simulink model "CL_NL_DH_GUIA_Original"  (R2025b)
settings: Solver=ode4  StartTime=0.0  StopTime=200  FixedStep=Ts  RelTol=1e-3
values from neighbouring files (symbols this model uses):
  alpha_prot = deg2rad(16)    [guiagem_NL.m]
  att_alt = 0    [guiagem_NL.m]
  de_trim = U_trim(2)    [guiagem_NL.m]
  h0 = 600    [guiagem_NL.m]
  h_ref0 = h0    (= 600)    [guiagem_NL.m]
  i = find([Plantas.Ve] == VT_missao & [Plantas.He] == 600, 1)    [guiagem_NL.m]
  K_bank_guia = 0.1975    [guiagem_NL.m]
  phi_max_guia = deg2rad(20)    [guiagem_NL.m]
  phi_psi = 0    [guiagem_NL.m]
  prot_on = 0    [guiagem_NL.m]
  sat_surf_rad = deg2rad(sat_deg)    [guiagem_NL.m]
  surfaces = 24    [guiagem_NL.m]
  U_trim = double(Plantas(i).Ue(1:4))    [guiagem_NL.m]
  VT_ref0 = VT_missao    [guiagem_NL.m]
  VT_Throttle = 1    [guiagem_NL.m]
  WPs = [ 256    0  600  15 ... (first row only)    [guiagem_NL.m]
  xi_alt0 = double(Plantas(i).Xe(8)) / double(GintLong_Alt{i})    [guiagem_NL.m]
undefined symbols (not defined in the file or in its folder): act, eng, Plantas, R_accept, TrimInput
libraries: simulink_extras x10, simulink x1
settings Model: SimulationMode=accelerator  Creator=mirko  LastModifiedBy=mirko

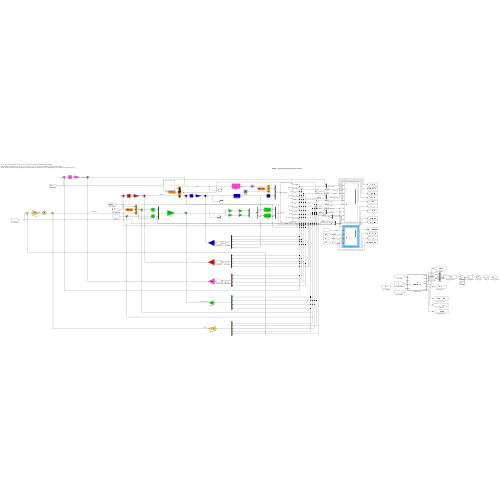
[thumbnail: Simulink's stored preview of the top-level diagram]
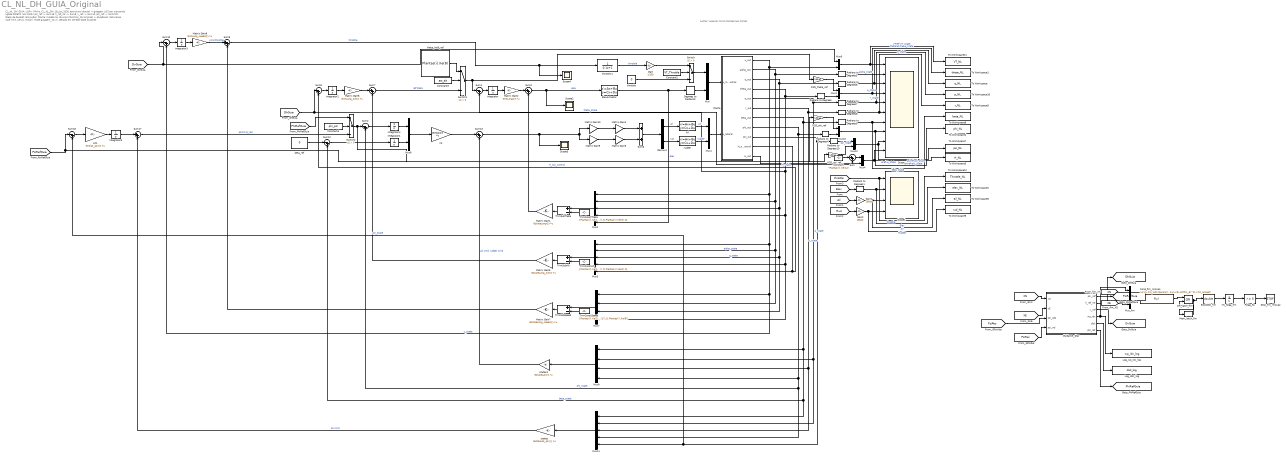
== system CL_NL_DH_GUIA_Original ==
  note: Author: Huascar Mirko Montecinos Cortez
  note: CL_NL_DH_GUIA: LQRy (Mirko, CL_NL_DH_18_jun_2026, estrutura intacta) + guiagem LOS por waypoints
      | ligada DIRETO nos holds (psi_ref -> Sum18, h_ref_rel -> Sum8, v_ref -> Sum10, phi_ref -> Switch2). Steps de doublet removidos.
      | Planta: modelo NL da Ana (sfunction_DH original) + atuadores (saturacao, rate limit, servo, motor). Rode guiagem_NL.m. Gerado em 03-Sep-2026 14:46:32.
  Ail : StateSpace  A=-surfaces  B=surfaces  D=0  InitialCondition=0
  Bool2Dbl_fim : DataTypeConversion  OutDataTypeStr=double  SaturateOnIntegerOverflow=off  RndMeth=Floor
  Cond_fim_missao : Fcn  Expr=(u(1)>=N_WPs)&&(sqrt((u(2)-WPfim_N)^2+(u(3)-WPfim_E)^2)<=R_accept)
  Constant : Constant  Value=-Plantas(i).Xe(12)
  Constant2 : Constant  Value=VT_Throttle
  Constant3 : Constant  Value=att_alt
  Constant4 : Constant  Value=phi_psi
  Degrees to Radians3 : simulink_extras/Transformations/Degrees to Radians
  Demux4 : Demux  Outputs=2
      settings: DisplayOption=none
  ElevActuator : StateSpace  A=-surfaces  B=surfaces  D=0  InitialCondition=Plantas(i).Ue(2)
  Folga_5s : simulink/Logic and Bit Operations/Compare To Constant  relop=>=  const=5  OutDataTypeStr=boolean
  Gain : Gain  Gain=1/100
  Gain1 : Gain  Gain=180/pi
  Gain2 : Gain  Gain=180/pi
  Guidance_Star : MATLAB Function  TreatAsAtomicUnit=on
  Int_folga_fim : Integrator
  Integrator{,1,3..5} (5 alike) : Integrator
  Integrator2 : Integrator  InitialCondition=xi_alt0
  Log_dist_log : ToWorkspace  VariableName=dist_log  SampleTime=-1
  Log_wp_idx_log : ToWorkspace  VariableName=wp_idx_log  SampleTime=-1
  Matrix Gain1 : Gain  Gain=GstateLong{i}  Multiplication=Matrix(K*u)  SaturateOnIntegerOverflow=on  OutDataTypeStr=Inherit: Same as input  ParamDataTypeStr=Inherit: Same as input
  Matrix Gain10 : Gain  Gain=[1 0]  Multiplication=Matrix(K*u)  SaturateOnIntegerOverflow=on  OutDataTypeStr=Inherit: Same as input  ParamDataTypeStr=Inherit: Same as input
  Matrix Gain2 : Gain  Gain=GintLong{i}  Multiplication=Matrix(K*u)  SaturateOnIntegerOverflow=on  OutDataTypeStr=Inherit: Same as input  ParamDataTypeStr=Inherit: Same as input
  Matrix Gain3 : Gain  Gain=[0 1]'  Multiplication=Matrix(K*u)  SaturateOnIntegerOverflow=on  OutDataTypeStr=Inherit: Same as input  ParamDataTypeStr=Inherit: Same as input
  Matrix Gain4 : Gain  Gain=[1 0]'  Multiplication=Matrix(K*u)  SaturateOnIntegerOverflow=on  OutDataTypeStr=Inherit: Same as input  ParamDataTypeStr=Inherit: Same as input
  Matrix Gain5 : Gain  Gain=GstateLong_Alt{i}  Multiplication=Matrix(K*u)  SaturateOnIntegerOverflow=on  OutDataTypeStr=Inherit: Same as input  ParamDataTypeStr=Inherit: Same as input
  Matrix Gain6 : Gain  Gain=GintLong_Alt{i}  Multiplication=Matrix(K*u)  SaturateOnIntegerOverflow=on  OutDataTypeStr=Inherit: Same as input  ParamDataTypeStr=Inherit: Same as input
  Matrix Gain7 : Gain  Gain=GstateLong_speed{i}  Multiplication=Matrix(K*u)  SaturateOnIntegerOverflow=on  OutDataTypeStr=Inherit: Same as input  ParamDataTypeStr=Inherit: Same as input
  Matrix Gain8 : Gain  Gain=GintLong_speed{i}  Multiplication=Matrix(K*u)  SaturateOnIntegerOverflow=on  OutDataTypeStr=Inherit: Same as input  ParamDataTypeStr=Inherit: Same as input
  Matrix Gain9 : Gain  Gain=[0 1]  Multiplication=Matrix(K*u)  SaturateOnIntegerOverflow=on  OutDataTypeStr=Inherit: Same as input  ParamDataTypeStr=Inherit: Same as input
  Mem_latch_fim : Memory
  Mux{,1,3..4,6,8,10,12} (8 alike) : Mux  Inputs=2
  Mux11 : Mux  Inputs=5
  Mux2 : Mux  Inputs=5
  Mux5 : Mux  Inputs=5
  Mux7 : Mux
  Mux9 : Mux
  Mux_fim : Mux  Inputs=3
  OR_latch_fim : Logic  Operator=OR  AllPortsSameDT=off  OutDataTypeStr=boolean
  Planta : Subsystem
  R2D_phi_ref : Gain  Gain=180/pi
  R2D_psi_ref : Gain  Gain=180/pi
  R2D_theta_ref : Gain  Gain=180/pi
  Radians to Degrees{,1,4..10} (9 alike) : simulink_extras/Transformations/Radians to Degrees
  Scope : Scope  NumInputPorts=10
      settings: ActiveDisplayString=10  ActiveDisplayYMinimum=599.95100767099655  ActiveDisplayYMaximum=600.03459621742491
  Scope1 : Scope  NumInputPorts=4
      settings: ActiveDisplayString=4  ActiveDisplayYMinimum=-3.1238215479894382  ActiveDisplayYMaximum=4.435550961328742
  Scope2 : Scope
      settings: ActiveDisplayYMinimum=-1.3531942213324573  ActiveDisplayYMaximum=0.61662907005096645  DataLoggingVariableName=ScopeData2
  Scope3 : Scope
      settings: ActiveDisplayYMinimum=-0.008953837623387962  ActiveDisplayYMaximum=0.0080763644870395709  DataLoggingVariableName=ScopeData3
  Scope4 : Scope
      settings: ActiveDisplayYMinimum=-268.65761065429206  ActiveDisplayYMaximum=1519.894817061396  DataLoggingVariableName=ScopeData4
  Stop_fim_missao : Stop
  Sum{,3,7,9} (4 alike) : Sum  Inputs=|++
  Sum1 : Sum  Inputs=|-+
  Sum10 : Sum  Inputs=|-+
  Sum12 : Sum  Inputs=|-+  SaturateOnIntegerOverflow=on
  Sum13 : Sum  Inputs=|++  SaturateOnIntegerOverflow=on
  Sum17 : Sum  Inputs=|++  SaturateOnIntegerOverflow=on
  Sum18 : Sum  Inputs=|-+  SaturateOnIntegerOverflow=on
  Sum2 : Sum  Inputs=|-+  SaturateOnIntegerOverflow=on
  Sum6 : Sum  Inputs=2  SaturateOnIntegerOverflow=on
  Sum8 : Sum  Inputs=|-+
  Switch : Switch  Criteria=u2 > Threshold  SaturateOnIntegerOverflow=off  InputSameDT=off
  Switch1 : Switch  Criteria=u2 > Threshold  SaturateOnIntegerOverflow=off  InputSameDT=off
  Switch2 : Switch  Criteria=u2 > Threshold  SaturateOnIntegerOverflow=off  InputSameDT=off
  To Workspace : ToWorkspace  VariableName=q_NL  SaveFormat=Structure With Time  SampleTime=-1
  To Workspace1 : ToWorkspace  VariableName=theta_NL  SaveFormat=Structure With Time  SampleTime=-1
  To Workspace10 : ToWorkspace  VariableName=p_NL  SaveFormat=Structure With Time  SampleTime=-1
  To Workspace11 : ToWorkspace  VariableName=VT_NL  SaveFormat=Structure With Time  SampleTime=-1
  To Workspace12 : ToWorkspace  VariableName=Throttle_NL  SaveFormat=Structure With Time  SampleTime=-1
  To Workspace2 : ToWorkspace  VariableName=elev_NL  SaveFormat=Structure With Time  SampleTime=-1
  To Workspace3 : ToWorkspace  VariableName=H_NL  SaveFormat=Structure With Time  SampleTime=-1
  To Workspace4 : ToWorkspace  VariableName=phi_NL  SaveFormat=Structure With Time  SampleTime=-1
  To Workspace5 : ToWorkspace  VariableName=r_NL  SaveFormat=Structure With Time  SampleTime=-1
  To Workspace6 : ToWorkspace  VariableName=ail_NL  SaveFormat=Structure With Time  SampleTime=-1
  To Workspace7 : ToWorkspace  VariableName=psi_NL  SaveFormat=Structure With Time  SampleTime=-1
  To Workspace8 : ToWorkspace  VariableName=beta_NL  SaveFormat=Structure With Time  SampleTime=-1
  To Workspace9 : ToWorkspace  VariableName=rud_NL  SaveFormat=Structure With Time  SampleTime=-1
  TrimConstAlt : Constant  Value=[Plantas(i).Xe(1); atan(Plantas(i).Xe(3)/Plantas(i).Xe(1)); 0; Plantas(i).Xe(8); 0]  VectorParams1D=off
  TrimConstSpeed : Constant  Value=[Plantas(i).Xe(1); atan(Plantas(i).Xe(3)/Plantas(i).Xe(1)); 0; Plantas(i).Xe(8)]  VectorParams1D=off
  TrimConstTheta : Constant  Value=[Plantas(i).Xe(1); atan(Plantas(i).Xe(3)/Plantas(i).Xe(1)); 0; Plantas(i).Xe(8); 0]  VectorParams1D=off
  TrimSubAlt : Sum  Inputs=+-
  TrimSubSpeed : Sum  Inputs=+-
  TrimSubTheta : Sum  Inputs=+-
  beta_ref : Constant  Value=0
  int : Gain  Gain=Gintlat{i}  Multiplication=Matrix(K*u)  SaturateOnIntegerOverflow=on  OutDataTypeStr=Inherit: Same as input  ParamDataTypeStr=Inherit: Same as input
  int1 : Gain  Gain=Gintlat_psi{i}  Multiplication=Matrix(K*u)  SaturateOnIntegerOverflow=on  OutDataTypeStr=Inherit: Same as input  ParamDataTypeStr=Inherit: Same as input
  rudder : StateSpace  A=-surfaces  B=surfaces  D=0  InitialCondition=0
  states : Gain  Gain=GstateLat_psi{i}  Multiplication=Matrix(K*u)  SaturateOnIntegerOverflow=on  OutDataTypeStr=Inherit: Same as input  ParamDataTypeStr=Inherit: Same as input
  states1 : Gain  Gain=GstateLat{i}  Multiplication=Matrix(K*u)  SaturateOnIntegerOverflow=on  OutDataTypeStr=Inherit: Same as input  ParamDataTypeStr=Inherit: Same as input
  theta_hold_ref : Constant  Value=Plantas(i).Xe(8)
  throttle : Constant  Value=0
  throttle 1 : TransferFcn  Denominator=[0.1 1]
  tag scope: DhGuia=global, DvGuia=global, PhiRefGuia=global, PsiRefGuia=global
  wires:
  Mux/1 -> Planta/1(u_longitudinal)
  Mux1/1 -> Planta/2(u_lateral)
  Matrix Gain1/1 -> Sum3/2
  Matrix Gain2/1 -> Sum3/1
  Integrator/1 -> Matrix Gain2/1
  Sum1/1 -> Integrator/1
  Sum3/1 -> Scope2/1, ElevActuator/1  "elev"
  Planta/1(u_out) -> Mux6/2, Mux7/1, Sum10/2, Mux5/1, Mux2/1  "u_state"
  Planta/2(alpha_out) -> Mux7/2, Mux5/2, Mux2/2, Radians to Degrees5/1  "alpha_state"
  Planta/3(q_out) -> Mux7/3, Mux5/3, Mux2/3, Radians to Degrees6/1  "q_state"
  Planta/4(theta_out) -> Mux7/4, Mux5/4, Mux2/4, Sum1/2, Radians to Degrees/1  "theta_state"
  Planta/5(p_out) -> Radians to Degrees7/1, Mux9/2, Mux11/2  "p_state"
  Planta/6(r_out) -> Radians to Degrees8/1, Mux9/3, Mux11/3  "r_state"
  Planta/7(beta_out) -> Radians to Degrees9/1, Mux11/1, Sum12/2, Mux9/1  "beta_state"
  Planta/8(phi_out) -> Radians to Degrees4/1, Mux11/4, Sum2/2, Mux9/4  "phi_state"
  Planta/9(psi_out) -> Mux11/5, Sum18/2, Radians to Degrees10/1  "psi_state"
  Planta/10(H_out_control) -> Mux5/5, Sum8/2  "H_out_control"
  Mux3/1 -> To Workspace1/1, Scope/4  "thetaref-theta_state"
  Radians to Degrees/1 -> Mux3/2
  Matrix Gain5/1 -> Sum7/2
  Sum8/1 -> Integrator2/1
  Sum7/1 -> Switch1/3  "ref theta"
  Matrix Gain6/1 -> Sum7/1
  Integrator2/1 -> Matrix Gain6/1
  Mux4/1 -> Scope/10, To Workspace3/1  "Href-H_state"
  Constant/1 -> Sum/1
  Sum/1 -> Mux4/1
  Radians to Degrees1/1 -> Scope1/2, To Workspace2/1  "Elev"
  Gain1/1 -> Scope1/3, To Workspace6/1  "Ail"
  Gain2/1 -> Scope1/4, To Workspace9/1  "Rudder"
  Sum10/1 -> Integrator3/1
  Matrix Gain7/1 -> Sum9/2
  Integrator3/1 -> Matrix Gain8/1
  Matrix Gain8/1 -> Sum9/1  "cmd throttle"
  [Elev] -> Radians to Degrees1/1
  [Ail] -> Gain1/1
  [Rud] -> Gain2/1
  [throttle] -> To Workspace12/1, Scope1/1  "throttle"
  Sum9/1 -> Scope4/1, throttle 1/1  "throttle"
  Mux6/1 -> To Workspace11/1, Scope/1  "VTref-VT_state"
  Matrix Gain9/1 -> Matrix Gain3/1
  Matrix Gain10/1 -> Matrix Gain4/1
  Matrix Gain4/1 -> Sum6/1
  Sum13/1 -> Scope3/1, Matrix Gain9/1, Matrix Gain10/1
  Matrix Gain3/1 -> Sum6/2
  Sum6/1 -> Demux4/1
  Demux4/2 -> rudder/1  "rud"
  Demux4/1 -> Ail/1  "ail"
  int/1 -> Sum13/1
  Mux8/1 -> int/1
  Sum12/1 -> Integrator1/1
  Integrator4/1 -> Mux8/1
  Integrator1/1 -> Mux8/2
  Sum2/1 -> Integrator4/1
  Mux9/1 -> states1/1
  states1/1 -> Sum13/2  "ail cmd, rudder cmd"
  Mux10/1 -> To Workspace4/1, Scope/8  "phiref-phi_state"
  Radians to Degrees4/1 -> Mux10/2
  throttle/1 -> Switch/3
  Radians to Degrees5/1 -> Scope/2  "alpha_state"
  Radians to Degrees6/1 -> To Workspace/1, Scope/3  "q_state"
  Radians to Degrees7/1 -> To Workspace10/1, Scope/5  "p_state"
  Radians to Degrees8/1 -> Scope/6, To Workspace5/1  "r_state"
  Radians to Degrees9/1 -> Scope/7, To Workspace8/1  "beta_state"
  Degrees to Radians3/1 -> Mux/2
  Gain/1 -> Switch/1
  Mux12/1 -> To Workspace7/1, Scope/9  "psiref-psi_state"
  Planta/11(H_out) -> Mux4/2  "H_state"
  Mux11/1 -> states/1
  Sum18/1 -> int1/1
  Integrator5/1 -> Sum17/1
  int1/1 -> Integrator5/1
  Sum17/1 -> Switch2/3  "psiCmd_rad"
  states/1 -> Sum17/2  "ail cmd"
  Switch2/1 -> Sum2/1, R2D_phi_ref/1
  Radians to Degrees10/1 -> Mux12/1  "psi_state"
  Constant2/1 -> Switch/2
  Constant3/1 -> Switch1/2
  Constant4/1 -> Switch2/2
  Mux7/1 -> TrimSubSpeed/1
  TrimConstSpeed/1 -> TrimSubSpeed/2
  TrimSubSpeed/1 -> Matrix Gain7/1
  Mux2/1 -> TrimSubTheta/1
  TrimConstTheta/1 -> TrimSubTheta/2
  TrimSubTheta/1 -> Matrix Gain1/1
  Mux5/1 -> TrimSubAlt/1
  TrimConstAlt/1 -> TrimSubAlt/2
  TrimSubAlt/1 -> Matrix Gain5/1
  throttle 1/1 -> Gain/1  "throttle"
  rudder/1 -> Mux1/2  "rudder"
  Ail/1 -> Mux1/1  "Ail"
  ElevActuator/1 -> Degrees to Radians3/1, Mux2/5  "elev"
  Switch/1 -> Mux/1
  [XN] -> Guidance_Star/1(xN)
  [PsiRel] -> Guidance_Star/4(psi_rel)
  [PsiAbs] -> Guidance_Star/3(psi_abs)
  [XE] -> Guidance_Star/2(xE)
  Guidance_Star/1(psi_ref) -> [PsiRefGuia]
  Guidance_Star/2(h_ref_rel) -> [DhGuia]
  Guidance_Star/3(v_ref) -> [DvGuia]
  Guidance_Star/4(wp_idx) -> Log_wp_idx_log/1, Mux_fim/1
  Guidance_Star/5(dist) -> Log_dist_log/1
  Guidance_Star/6(phi_ref) -> [PhiRefGuia]
  [PsiRefGuia] -> Sum18/1, R2D_psi_ref/1
  [DhGuia] -> Sum8/1, Sum/2
  [DvGuia] -> Sum10/1, Mux6/1
  [PhiRefGuia] -> Switch2/1
  theta_hold_ref/1 -> Switch1/1
  Switch1/1 -> Sum1/1, R2D_theta_ref/1
  beta_ref/1 -> Sum12/1
  R2D_theta_ref/1 -> Mux3/1
  R2D_psi_ref/1 -> Mux12/2
  R2D_phi_ref/1 -> Mux10/1
  [XN] -> Mux_fim/2
  [XE] -> Mux_fim/3
  Mux_fim/1 -> Cond_fim_missao/1
  Cond_fim_missao/1 -> OR_latch_fim/1
  OR_latch_fim/1 -> Mem_latch_fim/1, Bool2Dbl_fim/1
  Mem_latch_fim/1 -> OR_latch_fim/2
  Bool2Dbl_fim/1 -> Int_folga_fim/1
  Int_folga_fim/1 -> Folga_5s/1
  Folga_5s/1 -> Stop_fim_missao/1

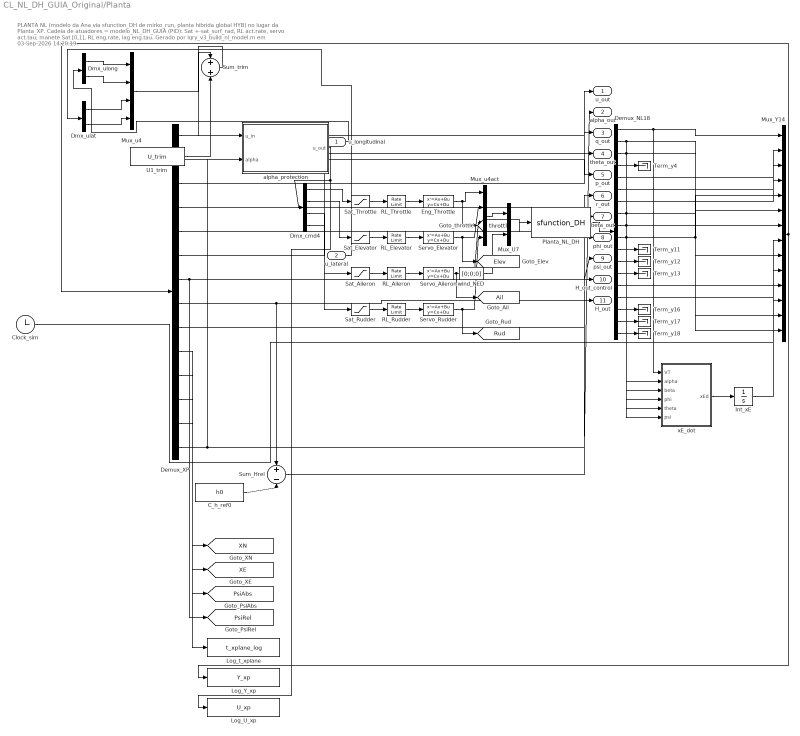
== system CL_NL_DH_GUIA_Original/Planta ==
  note: PLANTA NL (modelo da Ana via sfunction_DH de mirko_run, planta hibrida global HYB)
      | no lugar da Planta_XP. Cadeia de atuadores = modelo_NL_DH_GUIA (PID): Sat +-sat_surf_rad, RL act.rate,
      | servo act.tau; manete Sat [0,1], RL eng.rate, lag eng.tau. Gerado por lqry_v3_build_nl_model.m em 03-Sep-2026 14:20:19.
  u_longitudinal : Inport
  u_lateral : Inport  Port=2
  C_h_ref0 : Constant  Value=h0
  Clock_sim : Clock
  Demux_NL18 : Demux  Outputs=18
  Demux_XP : Demux  Outputs=14
  Dmx_cmd4 : Demux
  Dmx_ulat : Demux  Outputs=2
  Dmx_ulong : Demux  Outputs=2
  Eng_Throttle : StateSpace  A=-1/eng.tau  B=1/eng.tau  D=0  InitialCondition=U_trim(1)
  Int_xE : Integrator
  Log_U_xp : ToWorkspace  VariableName=U_xp  SampleTime=-1
  Log_Y_xp : ToWorkspace  VariableName=Y_xp  SampleTime=-1
  Log_t_xplane : ToWorkspace  VariableName=t_xplane_log  SampleTime=-1
  Mux_U7 : Mux  Inputs=2
  Mux_Y14 : Mux  Inputs=14
  Mux_u4 : Mux
  Mux_u4act : Mux
  Planta_NL_DH : S-Function  FunctionName=sfunction_DH  Parameters=Xe_planta, coef_Sato, coef_Ana, Variacao_Iner  SFunctionDeploymentMode=off  EnableBusSupport=off
  RL_Aileron : RateLimiter  RisingSlewLimit=act.rate  FallingSlewLimit=-act.rate  InitialCondition=TrimInput(3)
  RL_Elevator : RateLimiter  RisingSlewLimit=act.rate  FallingSlewLimit=-act.rate  InitialCondition=TrimInput(2)
  RL_Rudder : RateLimiter  RisingSlewLimit=act.rate  FallingSlewLimit=-act.rate  InitialCondition=TrimInput(4)
  RL_Throttle : RateLimiter  RisingSlewLimit=eng.rate  FallingSlewLimit=-eng.rate  InitialCondition=TrimInput(1)
  Sat_Aileron : Saturate  UpperLimit=sat_surf_rad  LowerLimit=-sat_surf_rad
  Sat_Elevator : Saturate  UpperLimit=sat_surf_rad  LowerLimit=-sat_surf_rad
  Sat_Rudder : Saturate  UpperLimit=sat_surf_rad  LowerLimit=-sat_surf_rad
  Sat_Throttle : Saturate  UpperLimit=1  LowerLimit=0
  Servo_Aileron : StateSpace  A=-act.bw  B=act.bw  D=0  InitialCondition=U_trim(3)
  Servo_Elevator : StateSpace  A=-act.bw  B=act.bw  D=0  InitialCondition=U_trim(2)
  Servo_Rudder : StateSpace  A=-act.bw  B=act.bw  D=0  InitialCondition=U_trim(4)
  Sum_Hrel : Sum  Inputs=+-
  Sum_trim : Sum
  Term_y{4,11..13,16..18} (7 alike) : Terminator
  U1_trim : Constant  Value=U_trim
  alpha_protection : MATLAB Function  TreatAsAtomicUnit=on
  wind_NED : Constant  Value=[0;0;0]
  xE_dot : MATLAB Function  TreatAsAtomicUnit=on
  u_out : Outport
  alpha_out : Outport  Port=2
  q_out : Outport  Port=3
  theta_out : Outport  Port=4
  p_out : Outport  Port=5
  r_out : Outport  Port=6
  beta_out : Outport  Port=7
  phi_out : Outport  Port=8
  psi_out : Outport  Port=9
  H_out_control : Outport  Port=10
  H_out : Outport  Port=11
  tag scope: Ail=global, Elev=global, PsiAbs=global, PsiRel=global, Rud=global, XE=global, XN=global, throttle=global
  wires:
  u_longitudinal/1 -> Dmx_ulong/1
  u_lateral/1 -> Dmx_ulat/1
  Dmx_ulong/1 -> Mux_u4/1
  Dmx_ulong/2 -> Mux_u4/2
  Dmx_ulat/1 -> Mux_u4/3
  Dmx_ulat/2 -> Mux_u4/4
  Demux_XP/1 -> u_out/1
  Demux_XP/14 -> alpha_out/1, alpha_protection/2(alpha)
  Demux_XP/3 -> q_out/1
  Demux_XP/6 -> theta_out/1
  Demux_XP/2 -> p_out/1
  Demux_XP/4 -> r_out/1
  Demux_XP/9 -> beta_out/1
  Demux_XP/5 -> phi_out/1
  Demux_XP/7 -> psi_out/1, [PsiRel]
  Demux_XP/8 -> Sum_Hrel/1, H_out/1
  C_h_ref0/1 -> Sum_Hrel/2
  Sum_Hrel/1 -> H_out_control/1
  Demux_XP/11 -> [XN]
  Demux_XP/12 -> [XE]
  Demux_XP/13 -> [PsiAbs]
  Demux_XP/10 -> Log_t_xplane/1
  Mux_u4/1 -> Sum_trim/1
  U1_trim/1 -> Sum_trim/2
  Sum_trim/1 -> alpha_protection/1(u_in)
  alpha_protection/1(u_out) -> Log_U_xp/1, Dmx_cmd4/1
  Dmx_cmd4/1 -> Sat_Throttle/1
  Sat_Throttle/1 -> RL_Throttle/1
  RL_Throttle/1 -> Eng_Throttle/1
  Dmx_cmd4/2 -> Sat_Elevator/1
  Sat_Elevator/1 -> RL_Elevator/1
  RL_Elevator/1 -> Servo_Elevator/1
  Dmx_cmd4/3 -> Sat_Aileron/1
  Sat_Aileron/1 -> RL_Aileron/1
  RL_Aileron/1 -> Servo_Aileron/1
  Dmx_cmd4/4 -> Sat_Rudder/1
  Sat_Rudder/1 -> RL_Rudder/1
  RL_Rudder/1 -> Servo_Rudder/1
  Eng_Throttle/1 -> Mux_u4act/1, [throttle]
  Servo_Elevator/1 -> Mux_u4act/2, [Elev]
  Servo_Aileron/1 -> Mux_u4act/3, [Ail]
  Servo_Rudder/1 -> Mux_u4act/4, [Rud]
  Mux_u4act/1 -> Mux_U7/1
  wind_NED/1 -> Mux_U7/2
  Mux_U7/1 -> Planta_NL_DH/1
  Planta_NL_DH/1 -> Demux_NL18/1
  Demux_NL18/4 -> Term_y4/1
  Demux_NL18/11 -> Term_y11/1
  Demux_NL18/12 -> Term_y12/1
  Demux_NL18/13 -> Term_y13/1
  Demux_NL18/16 -> Term_y16/1
  Demux_NL18/17 -> Term_y17/1
  Demux_NL18/18 -> Term_y18/1
  Demux_NL18/1 -> xE_dot/1(VT), Mux_Y14/1
  Demux_NL18/2 -> xE_dot/2(alpha), Mux_Y14/14
  Demux_NL18/3 -> xE_dot/3(beta), Mux_Y14/9
  Demux_NL18/8 -> xE_dot/4(phi), Mux_Y14/5
  Demux_NL18/9 -> xE_dot/5(theta), Mux_Y14/6
  Demux_NL18/10 -> Mux_Y14/7, Mux_Y14/13, xE_dot/6(psi)
  xE_dot/1(xEd) -> Int_xE/1
  Demux_NL18/5 -> Mux_Y14/2
  Demux_NL18/6 -> Mux_Y14/3
  Demux_NL18/7 -> Mux_Y14/4
  Demux_NL18/15 -> Mux_Y14/8
  Clock_sim/1 -> Mux_Y14/10
  Demux_NL18/14 -> Mux_Y14/11
  Int_xE/1 -> Mux_Y14/12
  Mux_Y14/1 -> Demux_XP/1, Log_Y_xp/1

== matlab function CL_NL_DH_GUIA_Original/Planta/xE_dot ==
  data: VT input; xEd output; alpha input; beta input; phi input; theta input; psi input
function xEd = xE_dot(VT, alpha, beta, phi, theta, psi)
% velocidade Leste inercial reconstruida das saidas do observador
% (exato p/ vento zero): [u v w] do triedro aerodinamico -> Lnb linha 2.
u = VT*cos(alpha)*cos(beta); v = VT*sin(beta); w = VT*sin(alpha)*cos(beta);
xEd = (sin(phi)*sin(theta)*sin(psi)+cos(phi)*cos(psi))*v ...
    + (cos(phi)*sin(theta)*sin(psi)-sin(phi)*cos(psi))*w ...
    + cos(theta)*sin(psi)*u;
end

== matlab function CL_NL_DH_GUIA_Original/Guidance_Star ==
  settings: updateMethod=DISCRETE  sampleTime=0.05
  data: xN input; psi_ref output; xE input; psi_abs input; psi_rel input; h_ref_rel output; v_ref output; wp_idx output; dist output; phi_ref output; WPs parameter; R_accept parameter; h_ref0 parameter; VT_ref0 parameter; K_bank_guia parameter; phi_max_guia parameter
function [psi_ref, h_ref_rel, v_ref, wp_idx, dist, phi_ref] = Guidance_Star(xN, xE, psi_abs, psi_rel, WPs, R_accept, h_ref0, VT_ref0, K_bank_guia, phi_max_guia)
% Guiagem LOS por waypoints (algoritmo do PIPER-1-6 do Julio, adaptado ao DH).
% Entradas: posicao xN/xE [m], proa absoluta psi_abs e relativa ao engate psi_rel [rad].
% WPs = [N E h V] (uma linha por waypoint); R_accept = raio de captura [m].
% Saidas (entram DIRETO nos holds do LQRy):
%   psi_ref   [rad] proa de referencia no mesmo referencial (relativo ao engate) que o psi Hold realimenta
%   h_ref_rel [m]   altitude do WP - h_ref0 (o Alt Hold trabalha com H relativa ao engate)
%   v_ref     [m/s] velocidade do WP (absoluta) -> Vel Hold
%   phi_ref   [rad] bank-to-turn, so' usado no modo phi Hold (phi_psi = 1); zero apos o ultimo WP
%   wp_idx, dist: monitor (WP alvo e distancia ate ele)
persistent k hold_fim
if isempty(k), k = 1; hold_fim = 0; end
n = size(WPs, 1); if k > n, k = n; end
dist = sqrt((WPs(k,1) - xN)^2 + (WPs(k,2) - xE)^2);
if dist <= R_accept
    if k < n, k = k + 1; else, hold_fim = 1; end
end
psi_los = atan2(WPs(k,2) - xE, WPs(k,1) - xN);
dpsi = mod(psi_los - psi_abs + pi, 2*pi) - pi;
psi_ref = psi_rel + dpsi;
if hold_fim, phi_ref = 0; else, phi_ref = min(max(K_bank_guia*dpsi, -phi_max_guia), phi_max_guia); end
h_ref_rel = WPs(k,3) - h_ref0;
v_ref = WPs(k,4) + 0*VT_ref0;
wp_idx = k;
end

== matlab function CL_NL_DH_GUIA_Original/Planta/alpha_protection ==
  settings: updateMethod=DISCRETE  sampleTime=0.05
  data: u_in input; u_out output; alpha input; prot_on parameter; alpha_prot parameter; de_trim parameter
function u_out = alpha_protection(u_in, alpha, prot_on, alpha_prot, de_trim)
% PROTECAO DE ENVELOPE DA PLATAFORMA (estilo fly-by-wire, 2026-08-30):
% quando alpha medido excede alpha_prot, o teto NOSE-UP do profundor
% desce em rampa (2 deg de alpha) ate o valor de trim — impede
% fisicamente a incursao de estol INDEPENDENTE do controlador.
% Implementada na Planta_XP (a "aeronave"), nao no controlador do
% Mirko: e' o unico jeito efetivo num regulador de estados (o clamp
% de referencia e' contornado pela realimentacao direta — testado).
u_out = u_in;
if prot_on > 0.5
    rampa = 2*pi/180;
    de_max_full = 25*pi/180;
    folga = alpha_prot - alpha;                % >0 abaixo do limite
    frac = min(1, max(0, folga/rampa));        % 1 = livre, 0 = so trim
    de_teto = de_trim + frac*(de_max_full - de_trim);
    u_out(2) = min(u_in(2), de_teto);
end
end
